simulink model "SP_Robot_AndroidApp"  (R2024a)
settings: Solver=VariableStepAuto  StartTime=0.0  StopTime=10.0  RelTol=1e-3
libraries: androidcommunicationlib x2, androiduilib x1, androidsensorlib x1, androidaudiovideolib x1
settings Model: Creator=ammaa  LastModifiedBy=ammaa

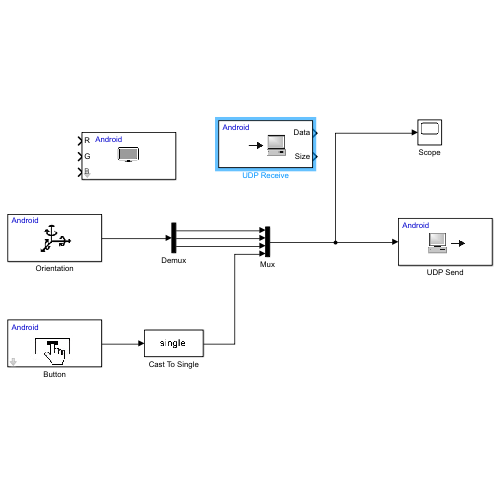
[thumbnail: Simulink's stored preview of the top-level diagram]
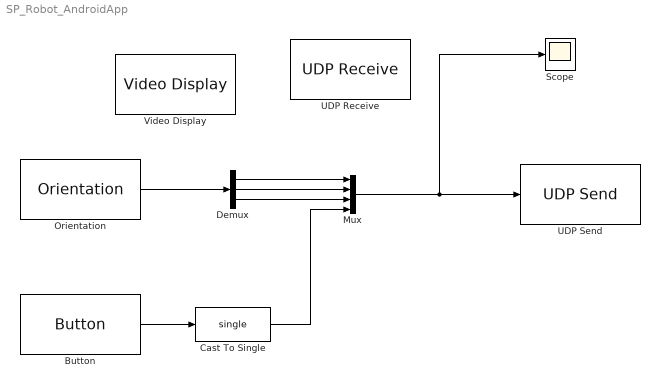
== system SP_Robot_AndroidApp ==
  Button : androiduilib/Button  ButtonState=Not pressed  State=off  SampleTime=0.1  BlockPlatform=Android
  Cast To Single : DataTypeConversion  OutDataTypeStr=single  SaturateOnIntegerOverflow=off  RndMeth=Floor
  Demux : Demux  Outputs=3
  Mux : Mux
  Orientation : androidsensorlib/Orientation  SampleTime=0.1
  Scope : Scope
  UDP Receive : androidcommunicationlib/UDP Receive  localURL='0.0.0.0'  localPort=25000  remoteURL='0.0.0.0'  remotePort=-1  recvBufferSize=8192  signalDatatype=uint8  dims=255  isVarSize=off  showBlockingTime=off  blockingTime=0  sampletime=0.01  blockPlatform=Android
  UDP Send : androidcommunicationlib/UDP Send  remoteURL='255.255.255.255'  remotePort=25000  localURL='0.0.0.0'  localPortSource=Automatically determine  localPort=-1  sampletime=-1  blockPlatform=Android  separateLengthPort=0
  Video Display : androidaudiovideolib/Video Display  BlockPlatform=Android
  wires:
  Orientation/1 -> Demux/1
  Mux/1 -> Scope/1, UDP Send/1
  Demux/1 -> Mux/1
  Demux/2 -> Mux/2
  Demux/3 -> Mux/3
  Button/1 -> Cast To Single/1
  Cast To Single/1 -> Mux/4
